simulink library "MagicFormulaTyreLibrary"  (R2021a)
settings: Solver=VariableStepAuto  StartTime=0.0  StopTime=10.0  RelTol=1e-3
settings Model: Creator=Tom  LastModifiedBy=Tom

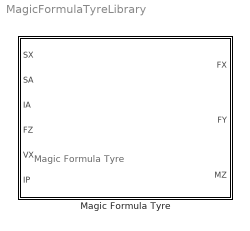
== system MagicFormulaTyreLibrary ==
  note: Magic Formula Tyre
  Magic Formula Tyre : Subsystem  mask(Magic Formula Tyre){file='doc/examples/fsae-ttc-data/fsaettc_obfuscated.tir', p=struct(), usemode=0}
      mask prompts: file "TIR file"; usemode "Mounting side (LEFT=0, RIGHT=1)"
      mask help: Evaluates Magic Formula (6.1.2) parameters
      mask init:
      | tyremodel = magicformula.v62.Model(file);
      | p = tyremodel.Parameters;
      | p = struct(p);
      | % set_param(gcb(), 'p', 'p');
      mask Help: https://github.com/teasit/magic-formula-tyre-library
      mask Display: image('MFTyreLibrary_PackageImage.png'); % Use "Edit Image" on toolstrip to change.

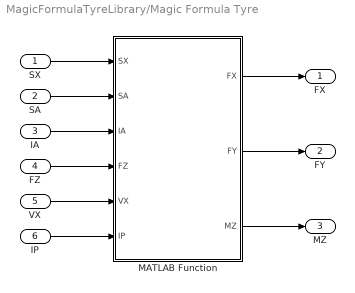
== system MagicFormulaTyreLibrary/Magic Formula Tyre ==
  SX : Inport  Unit=1
  SA : Inport  Port=2  Unit=rad
  IA : Inport  Port=3  Unit=rad
  FZ : Inport  Port=4  Unit=N
  VX : Inport  Port=5  Unit=m/s
  IP : Inport  Port=6  Unit=Pa
  MATLAB Function : MATLAB Function  TreatAsAtomicUnit=on
  FX : Outport  Unit=N
  FY : Outport  Port=2  Unit=N
  MZ : Outport  Port=3  Unit=N*m
  wires:
  SX/1 -> MATLAB Function/1(SX)
  MATLAB Function/1(FX) -> FX/1
  MATLAB Function/2(FY) -> FY/1
  MATLAB Function/3(MZ) -> MZ/1
  SA/1 -> MATLAB Function/2(SA)
  IA/1 -> MATLAB Function/3(IA)
  FZ/1 -> MATLAB Function/4(FZ)
  VX/1 -> MATLAB Function/5(VX)
  IP/1 -> MATLAB Function/6(IP)

== matlab function MagicFormulaTyreLibrary/Magic Formula Tyre/MATLAB Function ==
  data: FX output; p parameter size=1; SX input; SA input; IA input; FZ input; VX input; IP input; FY output; MZ output; usemode parameter
function [FX,FY,MZ] = eval(p,SX,SA,IA,FZ,VX,IP,usemode)
[FX,FY,MZ] = magicformula.v62.eval(p,SX,SA,IA,FZ,VX,IP,usemode);
